simulink model "zad1"  (R2021b)
settings: Solver=ode45  StartTime=0.0  StopTime=30.0  MaxStep=0.01  RelTol=1e-3
settings Model: Creator=Studenci  LastModifiedBy=Studenci

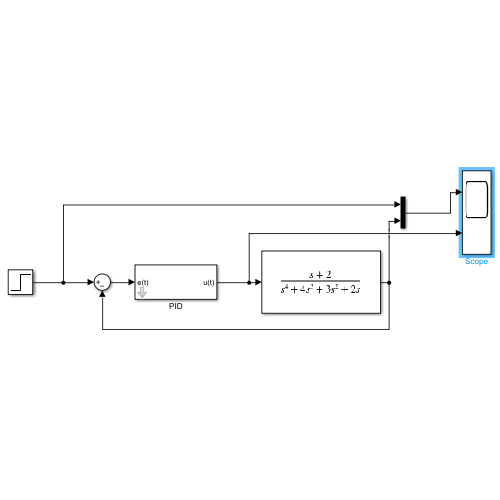
[thumbnail: Simulink's stored preview of the top-level diagram]
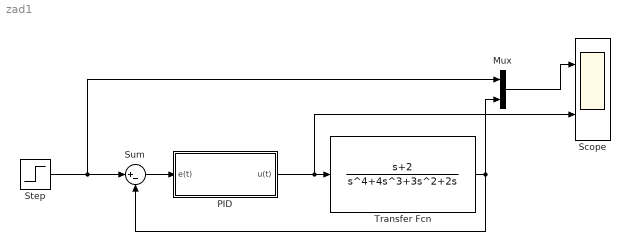
== system zad1 ==
  Mux : Mux  Inputs=2
  PID : Subsystem  mask{Kp=1, Ki=0, Kd=0}
      mask prompts: Kp "Kp ="; Ki "Ki ="; Kd "Kd ="
  Scope : Scope  NumInputPorts=2
  Step : Step  Time=0  SampleTime=0
  Sum : Sum  Inputs=|+-
  Transfer Fcn : TransferFcn  Numerator=[1 2]  Denominator=[1 4 3 2 0]
  wires:
  Sum/1 -> PID/1(e(t))
  Step/1 -> Mux/1, Sum/1
  PID/1(u(t)) -> Scope/2, Transfer Fcn/1
  Mux/1 -> Scope/1
  Transfer Fcn/1 -> Sum/2, Mux/2

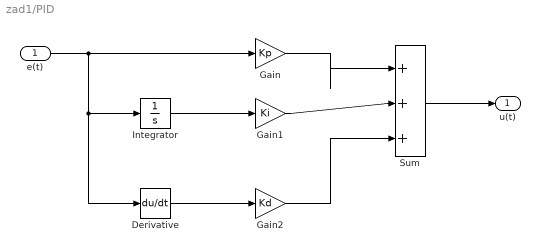
== system zad1/PID ==
  e(t) : Inport
  Derivative : Derivative
  Gain : Gain  Gain=Kp
  Gain1 : Gain  Gain=Ki
  Gain2 : Gain  Gain=Kd
  Integrator : Integrator
  Sum : Sum  Inputs=|+++
  u(t) : Outport
  wires:
  e(t)/1 -> Derivative/1, Integrator/1, Gain/1
  Gain/1 -> Sum/1
  Integrator/1 -> Gain1/1
  Derivative/1 -> Gain2/1
  Gain2/1 -> Sum/3
  Gain1/1 -> Sum/2
  Sum/1 -> u(t)/1
